simulink model "tank_system_simulink"  (R2019b)
settings: Solver=VariableStepAuto  StartTime=0.0  StopTime=10  RelTol=1e-3
settings Model: Creator=Δημήτρης  LastModifiedBy=Εμμανουήλ

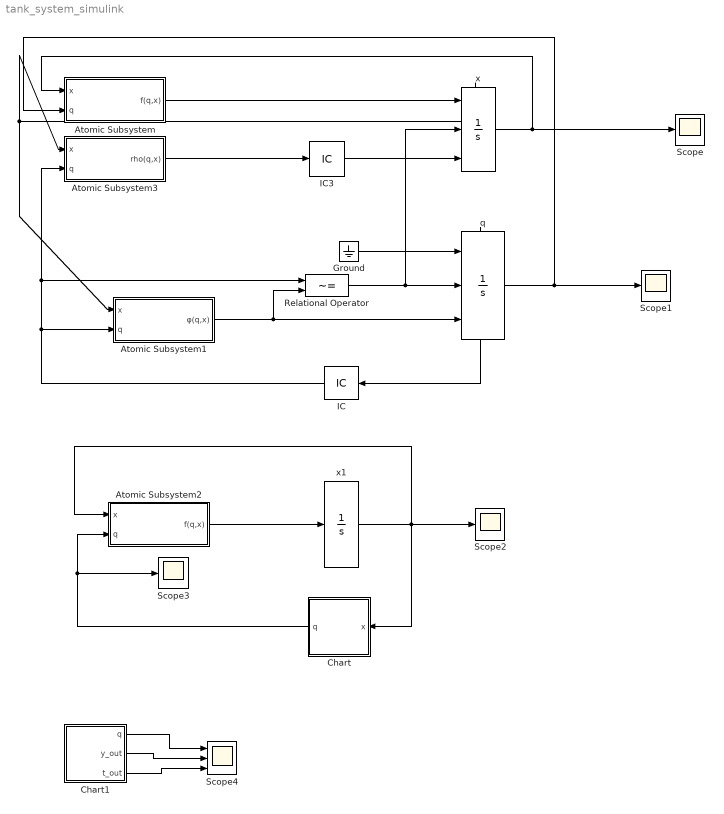
== system tank_system_simulink ==
  Atomic Subsystem : Subsystem  TreatAsAtomicUnit=on
  Atomic Subsystem1 : Subsystem  TreatAsAtomicUnit=on
  Atomic Subsystem2 : Subsystem  TreatAsAtomicUnit=on
  Atomic Subsystem3 : Subsystem  TreatAsAtomicUnit=on
  Chart : Stateflow chart  BlockKeywords=__PRM__SERIALIZED__DATA__:Stateflow Chart,Stateflow Diagram  TreatAsAtomicUnit=on
  Chart1 : Stateflow chart  BlockKeywords=__PRM__SERIALIZED__DATA__:Stateflow Chart,Stateflow Diagram  TreatAsAtomicUnit=on
  Ground : Ground
  IC : InitialCondition  Value=[1]
  IC3 : InitialCondition  Value=[4;0]
  Relational Operator : RelationalOperator  Operator=~=  OutDataTypeStr=boolean  RndMeth=Simplest
  Scope{,1..3} (4 alike) : Scope
  Scope4 : Scope  NumInputPorts=3
  q : Integrator  ExternalReset=rising  InitialConditionSource=external  ShowStatePort=on
  x : Integrator  ExternalReset=rising  InitialConditionSource=external  ShowStatePort=on
  x1 : Integrator  InitialCondition=[4]
  wires:
  Ground/1 -> q/1
  q/State -> IC/1
  IC/1 -> Atomic Subsystem3/2(q), Relational Operator/1, Atomic Subsystem1/2(q)
  Relational Operator/1 -> q/2, x/2
  q/1 -> Scope1/1, Atomic Subsystem/2(q)
  x/1 -> Atomic Subsystem/1(x), Scope/1
  Atomic Subsystem/1("f(q,x) ") -> x/1
  Atomic Subsystem1/1(φ(q,x)) -> q/3, Relational Operator/2
  x/State -> Atomic Subsystem3/1(x), Atomic Subsystem1/1(x)
  IC3/1 -> x/3
  Atomic Subsystem3/1("rho(q,x) ") -> IC3/1
  Chart/1(q) -> Atomic Subsystem2/2(q), Scope3/1
  x1/1 -> Chart/1(x), Scope2/1, Atomic Subsystem2/1(x)
  Atomic Subsystem2/1("f(q,x) ") -> x1/1
  Chart1/1(q) -> Scope4/1
  Chart1/2(y_out) -> Scope4/2
  Chart1/3(t_out) -> Scope4/3

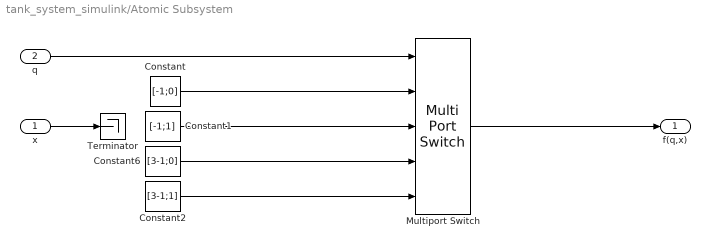
== system tank_system_simulink/Atomic Subsystem ==
  x : Inport
  q : Inport  Port=2
  Constant : Constant  Value=[-1;0]
  Constant1 : Constant  Value=[-1;1]
  Constant2 : Constant  Value=[3-1;1]
  Constant6 : Constant  Value=[3-1;0]
  Multiport Switch : MultiPortSwitch  Inputs=4
  Terminator : Terminator
  "f(q,x) " : Outport
  wires:
  x/1 -> Terminator/1
  q/1 -> Multiport Switch/1
  Multiport Switch/1 -> "f(q,x) "/1
  Constant1/1 -> Multiport Switch/3
  Constant6/1 -> Multiport Switch/4
  Constant/1 -> Multiport Switch/2
  Constant2/1 -> Multiport Switch/5

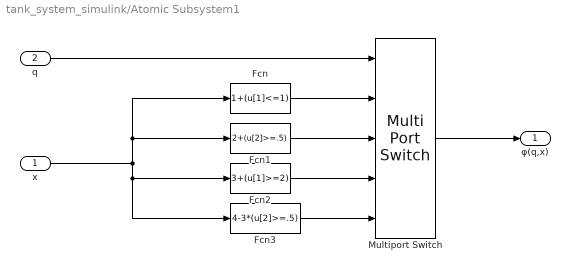
== system tank_system_simulink/Atomic Subsystem1 ==
  x : Inport
  q : Inport  Port=2
  Fcn : Fcn  Expr=1+(u[1]<=1)
  Fcn1 : Fcn  Expr=2+(u[2]>=.5)
  Fcn2 : Fcn  Expr=3+(u[1]>=2)
  Fcn3 : Fcn  Expr=4-3*(u[2]>=.5)
  Multiport Switch : MultiPortSwitch  Inputs=4
  φ(q,x) : Outport
  wires:
  Multiport Switch/1 -> φ(q,x)/1
  Fcn1/1 -> Multiport Switch/3
  Fcn/1 -> Multiport Switch/2
  x/1 -> Fcn1/1, Fcn/1, Fcn3/1, Fcn2/1
  q/1 -> Multiport Switch/1
  Fcn2/1 -> Multiport Switch/4
  Fcn3/1 -> Multiport Switch/5

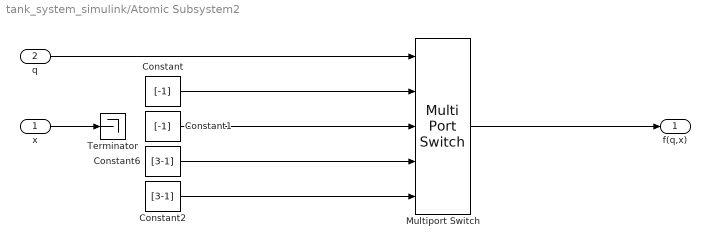
== system tank_system_simulink/Atomic Subsystem2 ==
  x : Inport
  q : Inport  Port=2
  Constant : Constant  Value=[-1]
  Constant1 : Constant  Value=[-1]
  Constant2 : Constant  Value=[3-1]
  Constant6 : Constant  Value=[3-1]
  Multiport Switch : MultiPortSwitch  Inputs=4
  Terminator : Terminator
  "f(q,x) " : Outport
  wires:
  Constant2/1 -> Multiport Switch/5
  Constant/1 -> Multiport Switch/2
  Constant6/1 -> Multiport Switch/4
  Constant1/1 -> Multiport Switch/3
  Multiport Switch/1 -> "f(q,x) "/1
  q/1 -> Multiport Switch/1
  x/1 -> Terminator/1

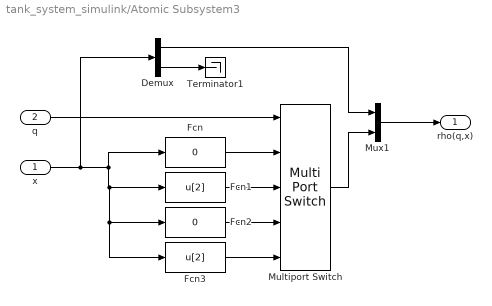
== system tank_system_simulink/Atomic Subsystem3 ==
  x : Inport
  q : Inport  Port=2
  Demux : Demux  Outputs=2
  Fcn : Fcn  Expr=0
  Fcn1 : Fcn  Expr=u[2]
  Fcn2 : Fcn  Expr=0
  Fcn3 : Fcn  Expr=u[2]
  Multiport Switch : MultiPortSwitch  Inputs=4
  Mux1 : Mux  Inputs=2
  Terminator1 : Terminator
  "rho(q,x) " : Outport
  wires:
  Fcn/1 -> Multiport Switch/2
  Fcn1/1 -> Multiport Switch/3
  q/1 -> Multiport Switch/1
  x/1 -> Demux/1, Fcn/1, Fcn3/1, Fcn2/1, Fcn1/1
  Mux1/1 -> "rho(q,x) "/1
  Multiport Switch/1 -> Mux1/2
  Fcn2/1 -> Multiport Switch/4
  Fcn3/1 -> Multiport Switch/5
  Demux/2 -> Terminator1/1
  Demux/1 -> Mux1/1

== stateflow chart tank_system_simulink/Chart1 ==
  settings: updateMethod=CONTINUOUS  executeAtInitialization=1  initializeOutput=1
  state pump_off
    du:
    y_dot = -1;
    t_dot = 0;
    q=1;
    y_out = y;
    t_out = t;
  state wait_to_off
    du:
    y_dot =3 -1;
    t_dot = 1;
    q=4;
    y_out = y;
    t_out = t;
  state pump_on
    du:
    y_dot = 3-1;
    t_dot = 0;
    q=3;
    y_out = y;
    t_out = t;
  state wait_to_on
    du:
    y_dot = -1;
    t_dot = 1;
    q=2;
    y_out = y;
    t_out = t;
  wait_to_off -> pump_off : after(0.5,sec)
  (default) -> pump_off : {y=4;t=0;}
  pump_off -> wait_to_on : [y<=1]{t=0}
  pump_on -> wait_to_off : [y>=3]{t=0}
  wait_to_on -> pump_on : after(0.5,sec)
  data: q output double size=1; y_out output double; t_out output double; t local double; y local double
  data t settings: updateMethod=SF_CONTINUOUS_TIME_DATA
  data y settings: updateMethod=SF_CONTINUOUS_TIME_DATA

== stateflow chart tank_system_simulink/Chart ==
  settings: updateMethod=CONTINUOUS
  state pump_off
    entry:q=1;
  state wait_to_off
    entry:q=4;
  state wait_to_on
    entry:q=2;
  state pump_on
    entry:q=3;
  wait_to_off -> pump_off : after(0.5,sec)
  (default) -> pump_off
  pump_off -> wait_to_on : [x(1)<=1]
  pump_on -> wait_to_off : [x(1)>=2]
  wait_to_on -> pump_on : after(0.5,sec)
  data: x input size=1; q output size=1
